simulink model "simulation"  (R2018a)
settings: Solver=VariableStepAuto  StartTime=0.0  StopTime=10.0  RelTol=1e-3
values from neighbouring files (symbols this model uses):
  b0 = 3    [taks.m]
  b1 = 3    [taks.m]
  K = 8    [taks.m]
settings Model: Creator=daniel  LastModifiedBy=daniel

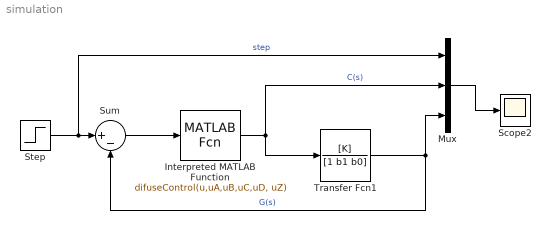
== system simulation ==
  Interpreted MATLAB Function : MATLABFcn  MATLABFcn=difuseControl(u,uA,uB,uC,uD, uZ)
  Mux : Mux  Inputs=3
  Scope2 : Scope
  Step : Step  SampleTime=0
  Sum : Sum  Inputs=|+-
  Transfer Fcn1 : TransferFcn  Numerator=[K]  Denominator=[1 b1 b0]
  wires:
  Transfer Fcn1/1 -> Mux/3, Sum/2  "G(s)"
  Step/1 -> Mux/1, Sum/1  "step"
  Interpreted MATLAB Function/1 -> Mux/2, Transfer Fcn1/1  "C(s)"
  Sum/1 -> Interpreted MATLAB Function/1
  Mux/1 -> Scope2/1
